simulink model "mainStateflow"  (R2020b)
settings: Solver=VariableStepAuto  StartTime=0.0  StopTime=86400  RelTol=1e-3
undefined symbols (not defined in the file or in its folder): m, n
libraries: SignalEditorBlockLib x1
settings Model: NumberOfSteps=5  Creator=Usuario  LastModifiedBy=Jesus Tapia

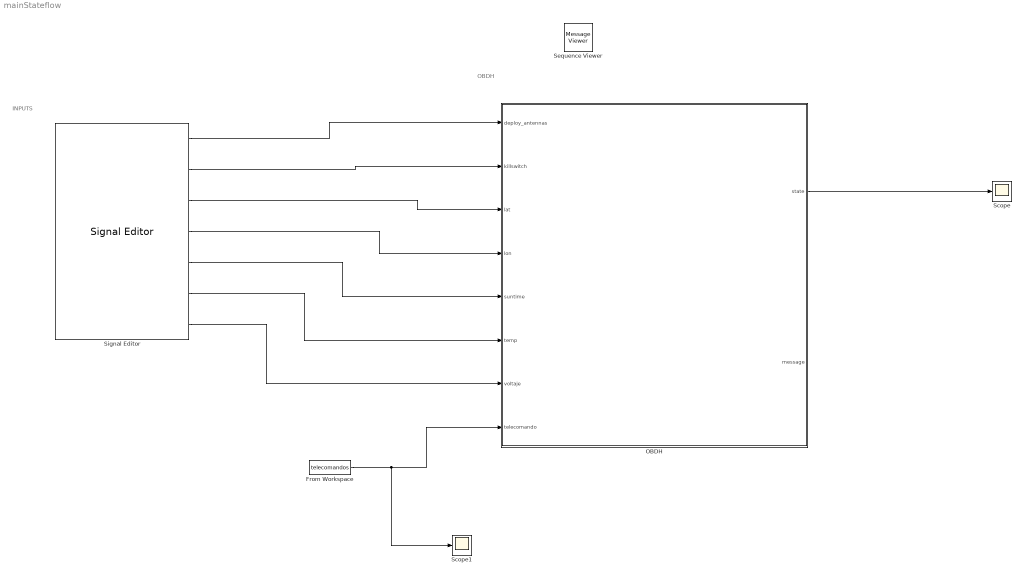
== system mainStateflow ==
  note: OBDH
  note: INPUTS
  From Workspace : FromWorkspace  VariableName=telecomandos
  OBDH : Stateflow chart  TreatAsAtomicUnit=on
  Scope : Scope
  Scope1 : Scope
  Sequence Viewer : MessageViewer
  Signal Editor : SignalEditorBlockLib/Signal Editor  FileName=main.mat  ActiveScenario=nominal  ActiveSignal=deploy_antennas  IsBus=off  OutputBusObjectStr=Bus: BusObject  SampleTime=0  Interpolate=off  ZeroCross=off  OutputAfterFinalValue=Setting to zero  Unit=inherit  PreserveSignalName=on
  wires:
  Signal Editor/7 -> OBDH/7(voltaje)
  Signal Editor/6 -> OBDH/6(temp)
  Signal Editor/1 -> OBDH/1(deploy_antennas)
  Signal Editor/2 -> OBDH/2(killswitch)
  Signal Editor/3 -> OBDH/3(lat)
  Signal Editor/4 -> OBDH/4(lon)
  Signal Editor/5 -> OBDH/5(suntime)
  OBDH/1(state) -> Scope/1
  From Workspace/1 -> Scope1/1, OBDH/8(telecomando)

== stateflow chart mainStateflow/OBDH ==
  state Off
    entry:
    state=0;
  state Boot
    entry:
    state=1;
    contBoot=1;
    during:
    contBoot=contBoot+1;
  state Safe
    entry:
    state=3;
  state Deploment
    entry:
    state=2;
    trydeploy=0;
    during:
    trydeploy=trydeploy+1;
  state Transmitiendo
    entry:
    state=5;
  state Nominal
    entry:
    state=4;
  (junction 78) -> (junction 82)
  (default) -> Off
  (junction 82) -> Off
  Safe -> (junction 78) [order 3] : [telecomando==0]
  Off -> Boot : [voltaje>5]
  Boot -> Deploment : [contBoot==360 || deploy_antennas==1]
  Nominal -> Off [order 2] : [telecomando==0]
  Deploment -> Off [order 2] : [telecomando==0]
  Deploment -> Safe [order 1] : [trydeploy==11 || deploy_antennas==1]
  Safe -> Nominal [order 1] : [telecomando==2]
  Nominal -> Safe [order 1] : [telecomando==3]
  Transmitiendo -> Safe [order 1] : [telecomando==3]
  Safe -> Transmitiendo [order 2] : [telecomando==4 & suntime==1]
  Transmitiendo -> Nominal [order 2] : [suntime==0]
  Nominal -> Transmitiendo [order 3] : [telecomando==4]
  data: deploy_antennas input; killswitch input; lat input; lon input; suntime input; temp input; v local; v1 local; voltaje input; state output; contBoot local; message output; trydeploy local; telecomando input; contOff local
